simulink model "Q7"  (R2016a)
settings: Solver=ode45  StartTime=0.0  StopTime=T  RelTol=1e-3
values from neighbouring files (symbols this model uses):
  b = 0    [e_11.m]    (also in e_12.m = 0.025; e_13.m; lab2.m)
  dy0 = dy    [e_11.m]    (also in lab2.m)
  y0 = y    [e_11.m]    (also in lab2.m)
settings Model: Creator=ricar  LastModifiedBy=ricar
settings DataIOCC: SaveFormat=Array
settings ModelReferenceCC: PropagateSignalLabelsOutOfModel=off

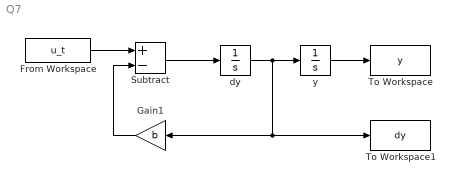
== system Q7 ==
  From Workspace : FromWorkspace  VariableName=u_t  SampleTime=0
  Gain1 : Gain  Gain=b
  Subtract : Sum  Inputs=+-
  To Workspace : ToWorkspace  VariableName=y  SampleTime=-1
  To Workspace1 : ToWorkspace  VariableName=dy  SampleTime=-1
  dy : Integrator  InitialCondition=dy0
  y : Integrator  InitialCondition=y0
  wires:
  From Workspace/1 -> Subtract/1
  Subtract/1 -> dy/1
  dy/1 -> To Workspace1/1, Gain1/1, y/1
  Gain1/1 -> Subtract/2
  y/1 -> To Workspace/1
